simulink model "PIDQUAD_Position"  (R2016a)
settings: Solver=ode4  StartTime=0.0  StopTime=14  FixedStep=0.01  RelTol=1e-3
undefined symbols (not defined in the file): Disturbance, g, Ix, Iy, Iz, Jr, L, m, omega
libraries: simulink x7
settings Model: Creator=Morteza  LastModifiedBy=Novin Pendar

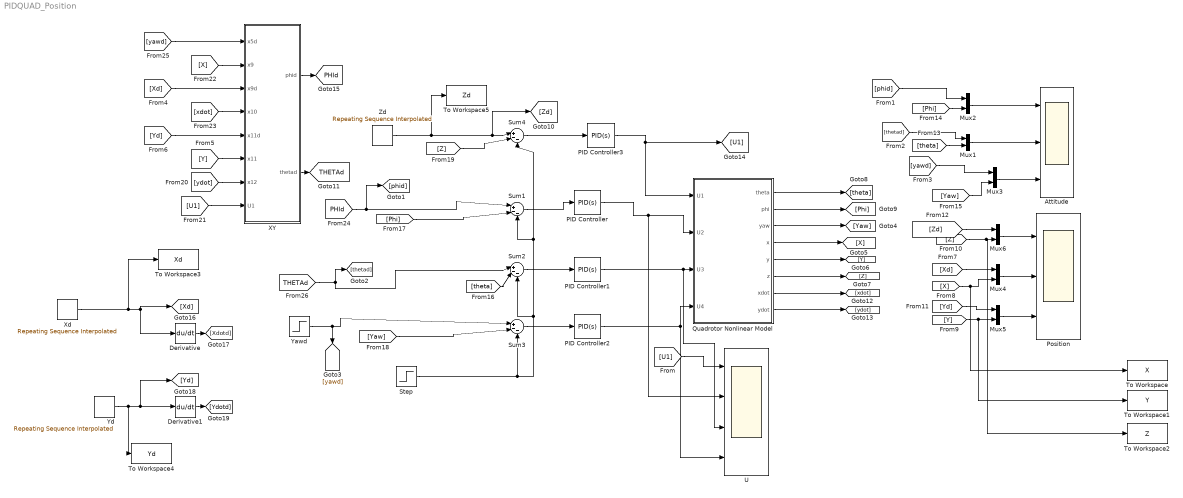
== system PIDQUAD_Position ==
  Attitude : Scope  NumInputPorts=3
  Derivative : Derivative
  Derivative1 : Derivative
  Mux{1..6} (6 alike) : Mux  Inputs=2
  PID Controller : simulink/Continuous/PID Controller  Controller=PID  TimeDomain=Continuous-time  SampleTime=-1  IntegratorMethod=Forward Euler  FilterMethod=Forward Euler  Form=Parallel  UseFilter=on  ControllerParametersSource=internal  P=5  I=1  D=0.199315858915149  N=100  InitialConditionSource=internal  InitialConditionForIntegrator=0  InitialConditionForFilter=0  ExternalReset=none  LimitOutput=off  UpperSaturationLimit=inf  LowerSaturationLimit=-inf  LinearizeAsGain=on  AntiWindupMode=none  Kb=1  TrackingMode=off  Kt=1  PParamMin=[]  PParamMax=[]  IParamMin=[]  IParamMax=[]  DParamMin=[]  DParamMax=[]  NParamMin=[]  NParamMax=[]  KbParamMin=[]  KbParamMax=[]  KtParamMin=[]  KtParamMax=[]  POutMin=[]  POutMax=[]  IOutMin=[]  IOutMax=[]  DOutMin=[]  DOutMax=[]  NOutMin=[]  NOutMax=[]  KbOutMin=[]  KbOutMax=[]  KtOutMin=[]  KtOutMax=[]  IntegratorOutMin=[]  IntegratorOutMax=[]  FilterOutMin=[]  FilterOutMax=[]  SumOutMin=[]  SumOutMax=[]  SumI1OutMin=[]  SumI1OutMax=[]  SumI2OutMin=[]  SumI2OutMax=[]  SumI3OutMin=[]  SumI3OutMax=[]  SumDOutMin=[]  SumDOutMax=[]  SaturationOutMin=[]  SaturationOutMax=[]  IntegratorContinuousStateAttributes=''  IntegratorStateMustResolveToSignalObject=off  IntegratorRTWStateStorageClass=Auto  FilterContinuousStateAttributes=''  FilterStateMustResolveToSignalObject=off  FilterRTWStateStorageClass=Auto  DifferentiatorICPrevScaledInput=0  DifferentiatorOutMin=[]  DifferentiatorOutMax=[]
  PID Controller1 : simulink/Continuous/PID Controller  Controller=PID  TimeDomain=Continuous-time  SampleTime=-1  IntegratorMethod=Forward Euler  FilterMethod=Forward Euler  Form=Parallel  UseFilter=on  ControllerParametersSource=internal  P=2  I=0.5  D=0.199315858915149  N=100  InitialConditionSource=internal  InitialConditionForIntegrator=0  InitialConditionForFilter=0  ExternalReset=none  LimitOutput=off  UpperSaturationLimit=inf  LowerSaturationLimit=-inf  LinearizeAsGain=on  AntiWindupMode=none  Kb=1  TrackingMode=off  Kt=1  PParamMin=[]  PParamMax=[]  IParamMin=[]  IParamMax=[]  DParamMin=[]  DParamMax=[]  NParamMin=[]  NParamMax=[]  KbParamMin=[]  KbParamMax=[]  KtParamMin=[]  KtParamMax=[]  POutMin=[]  POutMax=[]  IOutMin=[]  IOutMax=[]  DOutMin=[]  DOutMax=[]  NOutMin=[]  NOutMax=[]  KbOutMin=[]  KbOutMax=[]  KtOutMin=[]  KtOutMax=[]  IntegratorOutMin=[]  IntegratorOutMax=[]  FilterOutMin=[]  FilterOutMax=[]  SumOutMin=[]  SumOutMax=[]  SumI1OutMin=[]  SumI1OutMax=[]  SumI2OutMin=[]  SumI2OutMax=[]  SumI3OutMin=[]  SumI3OutMax=[]  SumDOutMin=[]  SumDOutMax=[]  SaturationOutMin=[]  SaturationOutMax=[]  IntegratorContinuousStateAttributes=''  IntegratorStateMustResolveToSignalObject=off  IntegratorRTWStateStorageClass=Auto  FilterContinuousStateAttributes=''  FilterStateMustResolveToSignalObject=off  FilterRTWStateStorageClass=Auto  DifferentiatorICPrevScaledInput=0  DifferentiatorOutMin=[]  DifferentiatorOutMax=[]
  PID Controller2 : simulink/Continuous/PID Controller  Controller=PID  TimeDomain=Continuous-time  SampleTime=-1  IntegratorMethod=Forward Euler  FilterMethod=Forward Euler  Form=Parallel  UseFilter=on  ControllerParametersSource=internal  P=0.417810086829264  I=0.2  D=0.347327554420679  N=34.4122258847421  InitialConditionSource=internal  InitialConditionForIntegrator=0  InitialConditionForFilter=0  ExternalReset=none  LimitOutput=off  UpperSaturationLimit=inf  LowerSaturationLimit=-inf  LinearizeAsGain=on  AntiWindupMode=none  Kb=1  TrackingMode=off  Kt=1  PParamMin=[]  PParamMax=[]  IParamMin=[]  IParamMax=[]  DParamMin=[]  DParamMax=[]  NParamMin=[]  NParamMax=[]  KbParamMin=[]  KbParamMax=[]  KtParamMin=[]  KtParamMax=[]  POutMin=[]  POutMax=[]  IOutMin=[]  IOutMax=[]  DOutMin=[]  DOutMax=[]  NOutMin=[]  NOutMax=[]  KbOutMin=[]  KbOutMax=[]  KtOutMin=[]  KtOutMax=[]  IntegratorOutMin=[]  IntegratorOutMax=[]  FilterOutMin=[]  FilterOutMax=[]  SumOutMin=[]  SumOutMax=[]  SumI1OutMin=[]  SumI1OutMax=[]  SumI2OutMin=[]  SumI2OutMax=[]  SumI3OutMin=[]  SumI3OutMax=[]  SumDOutMin=[]  SumDOutMax=[]  SaturationOutMin=[]  SaturationOutMax=[]  IntegratorContinuousStateAttributes=''  IntegratorStateMustResolveToSignalObject=off  IntegratorRTWStateStorageClass=Auto  FilterContinuousStateAttributes=''  FilterStateMustResolveToSignalObject=off  FilterRTWStateStorageClass=Auto  DifferentiatorICPrevScaledInput=0  DifferentiatorOutMin=[]  DifferentiatorOutMax=[]
  PID Controller3 : simulink/Continuous/PID Controller  Controller=PID  TimeDomain=Continuous-time  SampleTime=-1  IntegratorMethod=Forward Euler  FilterMethod=Forward Euler  Form=Parallel  UseFilter=on  ControllerParametersSource=internal  P=6  I=5  D=5  N=34.4122258847421  InitialConditionSource=internal  InitialConditionForIntegrator=0  InitialConditionForFilter=0  ExternalReset=none  LimitOutput=off  UpperSaturationLimit=inf  LowerSaturationLimit=-inf  LinearizeAsGain=on  AntiWindupMode=none  Kb=1  TrackingMode=off  Kt=1  PParamMin=[]  PParamMax=[]  IParamMin=[]  IParamMax=[]  DParamMin=[]  DParamMax=[]  NParamMin=[]  NParamMax=[]  KbParamMin=[]  KbParamMax=[]  KtParamMin=[]  KtParamMax=[]  POutMin=[]  POutMax=[]  IOutMin=[]  IOutMax=[]  DOutMin=[]  DOutMax=[]  NOutMin=[]  NOutMax=[]  KbOutMin=[]  KbOutMax=[]  KtOutMin=[]  KtOutMax=[]  IntegratorOutMin=[]  IntegratorOutMax=[]  FilterOutMin=[]  FilterOutMax=[]  SumOutMin=[]  SumOutMax=[]  SumI1OutMin=[]  SumI1OutMax=[]  SumI2OutMin=[]  SumI2OutMax=[]  SumI3OutMin=[]  SumI3OutMax=[]  SumDOutMin=[]  SumDOutMax=[]  SaturationOutMin=[]  SaturationOutMax=[]  IntegratorContinuousStateAttributes=''  IntegratorStateMustResolveToSignalObject=off  IntegratorRTWStateStorageClass=Auto  FilterContinuousStateAttributes=''  FilterStateMustResolveToSignalObject=off  FilterRTWStateStorageClass=Auto  DifferentiatorICPrevScaledInput=0  DifferentiatorOutMin=[]  DifferentiatorOutMax=[]
  Position : Scope  NumInputPorts=3
  Quadrotor Nonlinear Model : Subsystem
  Step : Step  Time=8  After=Disturbance  SampleTime=0
  Sum{1..4} (4 alike) : Sum  Inputs=|+--
  To Workspace : ToWorkspace  VariableName=X  SampleTime=-1
      settings: Save2DSignal=2-D array (concatenate along first dimension)
  To Workspace1 : ToWorkspace  VariableName=Y  SampleTime=-1
      settings: Save2DSignal=2-D array (concatenate along first dimension)
  To Workspace2 : ToWorkspace  VariableName=Z  SampleTime=-1
      settings: Save2DSignal=2-D array (concatenate along first dimension)
  To Workspace3 : ToWorkspace  VariableName=Xd  SampleTime=-1
      settings: Save2DSignal=2-D array (concatenate along first dimension)
  To Workspace4 : ToWorkspace  VariableName=Yd  SampleTime=-1
      settings: Save2DSignal=2-D array (concatenate along first dimension)
  To Workspace5 : ToWorkspace  VariableName=Zd  SampleTime=-1
      settings: Save2DSignal=2-D array (concatenate along first dimension)
  "U " : Scope  NumInputPorts=4
  XY : MATLAB Function  TreatAsAtomicUnit=on
  "Xd " : simulink/Sources/Repeating Sequence Interpolated  OutValues=[2 2 2 0 0].'  TimeValues="[0  3 6 9  14].'"  LookUpMeth=Interpolation-Use End Values  tsamp=0.01  OutMin=[]  OutMax=[]  OutDataTypeStr=double  OutputDataTypeScalingMode=double  OutDataType=fixdt(0,8)  OutScaling=2^-10
  Yawd : Step  Time=0  SampleTime=0
  "Yd " : simulink/Sources/Repeating Sequence Interpolated  OutValues=[2 2 5 5 0 0 ].'  TimeValues="[0 3  6 9 11 14].'"  LookUpMeth=Interpolation-Use End Values  tsamp=0.01  OutMin=[]  OutMax=[]  OutDataTypeStr=double  OutputDataTypeScalingMode=double  OutDataType=fixdt(0,8)  OutScaling=2^-10
  "Zd " : simulink/Sources/Repeating Sequence Interpolated  OutValues=[0.9 5 5].'  TimeValues="[0  3 14].'"  LookUpMeth=Interpolation-Use End Values  tsamp=0.01  OutMin=[]  OutMax=[]  OutDataTypeStr=double  OutputDataTypeScalingMode=double  OutDataType=fixdt(0,8)  OutScaling=2^-10
  tag scope: PHId=global, THETAd=global
  wires:
  Mux3/1 -> Attitude/3
  [thetad] -> Mux1/1
  [yawd] -> Mux3/1
  Quadrotor Nonlinear Model/5(y) -> [Y]
  Quadrotor Nonlinear Model/6(z) -> [Z]
  Quadrotor Nonlinear Model/4(x) -> [X]
  Quadrotor Nonlinear Model/3(yaw) -> [Yaw]
  Quadrotor Nonlinear Model/2(phi) -> [Phi]
  Quadrotor Nonlinear Model/1(theta) -> [theta]
  [Z] -> To Workspace2/1, Mux6/2
  [Y] -> To Workspace1/1, Mux5/2
  [X] -> To Workspace/1, Mux4/2
  [Zd] -> Mux6/1
  [Yd] -> Mux5/1
  [Xd] -> Mux4/1
  [theta] -> Mux1/2
  [Phi] -> Mux2/2
  [Yaw] -> Mux3/2
  Yawd/1 -> Sum3/1, [yawd]
  [Yaw] -> Sum3/2
  Sum1/1 -> PID Controller/1
  Sum2/1 -> PID Controller1/1
  Sum3/1 -> PID Controller2/1
  PID Controller/1 -> Quadrotor Nonlinear Model/2(U2), "U "/2
  PID Controller1/1 -> "U "/3, Quadrotor Nonlinear Model/3(U3)
  PID Controller2/1 -> Quadrotor Nonlinear Model/4(U4), "U "/4
  "Zd "/1 -> To Workspace5/1, [Zd], Sum4/1
  [Z] -> Sum4/2
  Sum4/1 -> PID Controller3/1
  PID Controller3/1 -> Quadrotor Nonlinear Model/1(U1), [U1]
  Mux1/1 -> Attitude/2
  Mux2/1 -> Attitude/1
  [Phi] -> Sum1/2
  [theta] -> Sum2/2
  Mux6/1 -> Position/1
  Mux4/1 -> Position/2
  Mux5/1 -> Position/3
  Quadrotor Nonlinear Model/7(xdot) -> [xdot]
  Quadrotor Nonlinear Model/8(ydot) -> [ydot]
  [THETAd] -> [thetad], Sum2/1
  [U1] -> "U "/1
  [phid] -> Mux2/1
  [X] -> XY/2(x9)
  [Xd] -> XY/3(x9d)
  [xdot] -> XY/4(x10)
  [Yd] -> XY/5(x11d)
  [Y] -> XY/6(x11)
  [ydot] -> XY/7(x12)
  [U1] -> XY/8(U1)
  XY/1(phid) -> [PHId]
  XY/2(thetad) -> [THETAd]
  [yawd] -> XY/1(x5d)
  "Xd "/1 -> To Workspace3/1, Derivative/1, [Xd]
  Derivative/1 -> [Xdotd]
  "Yd "/1 -> To Workspace4/1, [Yd], Derivative1/1
  Derivative1/1 -> [Ydotd]
  [PHId] -> Sum1/1, [phid]
  Step/1 -> Sum4/3, Sum1/3, Sum2/3, Sum3/3

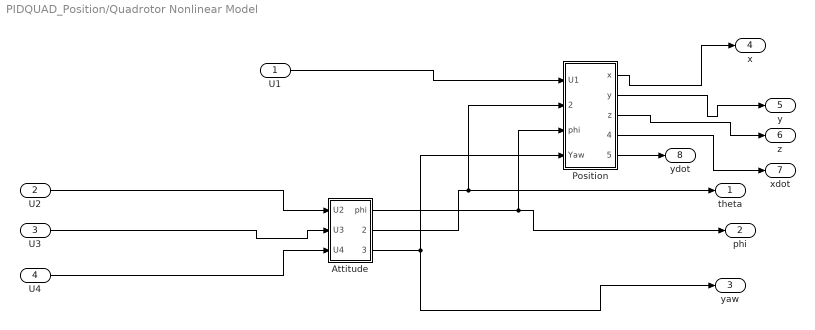
== system PIDQUAD_Position/Quadrotor Nonlinear Model ==
  U1 : Inport
  U2 : Inport  Port=2
  U3 : Inport  Port=3
  U4 : Inport  Port=4
  "Attitude " : Subsystem
  Position : Subsystem
  theta : Outport
  phi : Outport  Port=2
  yaw : Outport  Port=3
  x : Outport  Port=4
  y : Outport  Port=5
  z : Outport  Port=6
  xdot : Outport  Port=7
  ydot : Outport  Port=8
  wires:
  Position/2(y) -> y/1
  Position/3(z) -> z/1
  Position/1(x) -> x/1
  U3/1 -> "Attitude "/2(U3)
  U4/1 -> "Attitude "/3(U4)
  U2/1 -> "Attitude "/1(U2)
  "Attitude "/2(theta) -> Position/2(Theta), theta/1
  "Attitude "/1("phi ") -> Position/3(phi), phi/1
  U1/1 -> Position/1(U1)
  Position/4(xdot) -> xdot/1
  Position/5(ydot) -> ydot/1
  "Attitude "/3(yaw) -> yaw/1, Position/4(Yaw)

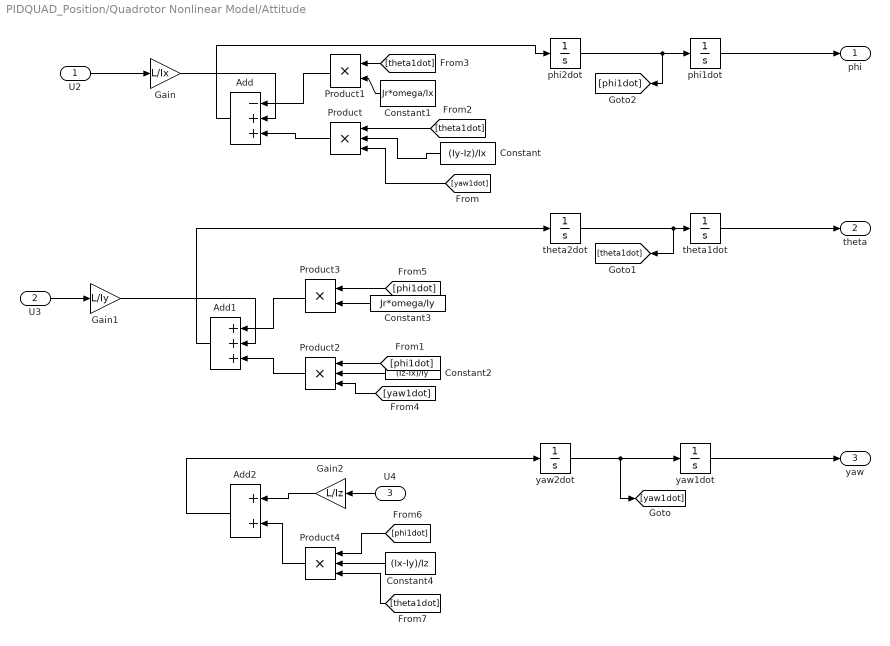
== system PIDQUAD_Position/Quadrotor Nonlinear Model/Attitude  ==
  U2 : Inport
  U3 : Inport  Port=2
  U4 : Inport  Port=3
  Add : Sum  Inputs=-++
  Add1 : Sum  Inputs=+++
  Add2 : Sum
  Constant : Constant  Value=(Iy-Iz)/Ix
  Constant1 : Constant  Value=Jr*omega/Ix
  Constant2 : Constant  Value=(Iz-Ix)/Iy
  Constant3 : Constant  Value=Jr*omega/Iy
  Constant4 : Constant  Value=(Ix-Iy)/Iz
  Gain : Gain  Gain=L/Ix
  Gain1 : Gain  Gain=L/Iy
  Gain2 : Gain  Gain=L/Iz
  Product : Product  Inputs=3
  Product1 : Product
  Product2 : Product  Inputs=3
  Product3 : Product
  Product4 : Product  Inputs=3
  phi1dot : Integrator
  phi2dot : Integrator
  theta1dot : Integrator
  theta2dot : Integrator
  yaw1dot : Integrator
  yaw2dot : Integrator
  "phi " : Outport
  theta : Outport  Port=2
  yaw : Outport  Port=3
  wires:
  theta2dot/1 -> [theta1dot], theta1dot/1
  Product/1 -> Add/3
  phi2dot/1 -> [phi1dot], phi1dot/1
  U2/1 -> Gain/1
  Add/1 -> phi2dot/1
  Product3/1 -> Add1/1
  [phi1dot] -> Product3/1
  Constant3/1 -> Product3/2
  U4/1 -> Gain2/1
  Product4/1 -> Add2/2
  Constant/1 -> Product/2
  Gain/1 -> Add/2
  phi1dot/1 -> "phi "/1
  yaw2dot/1 -> [yaw1dot], yaw1dot/1
  yaw1dot/1 -> yaw/1
  [yaw1dot] -> Product2/3
  Constant2/1 -> Product2/2
  [phi1dot] -> Product2/1
  Add2/1 -> yaw2dot/1
  Gain2/1 -> Add2/1
  [phi1dot] -> Product4/1
  [theta1dot] -> Product4/3
  Constant4/1 -> Product4/2
  Product2/1 -> Add1/3
  Product1/1 -> Add/1
  Add1/1 -> theta2dot/1
  U3/1 -> Gain1/1
  Gain1/1 -> Add1/2
  theta1dot/1 -> theta/1
  [theta1dot] -> Product/1
  [yaw1dot] -> Product/3
  Constant1/1 -> Product1/2
  [theta1dot] -> Product1/1

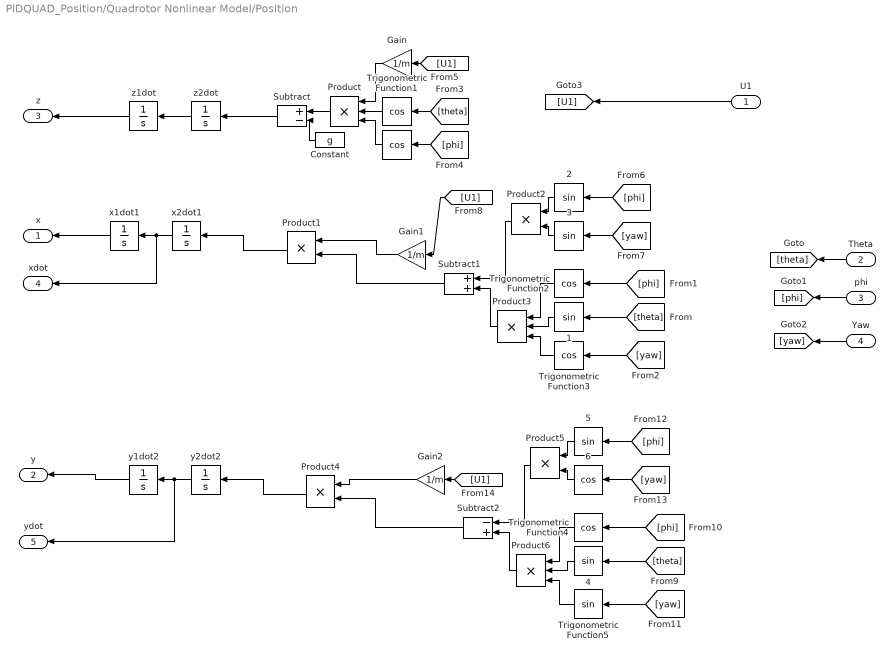
== system PIDQUAD_Position/Quadrotor Nonlinear Model/Position ==
  U1 : Inport
  Theta : Inport  Port=2
  phi : Inport  Port=3
  Yaw : Inport  Port=4
  " " : Trigonometry  Operator=cos
   {1..5} (5 alike) : Trigonometry
  " 6" : Trigonometry  Operator=cos
  Constant : Constant  Value=g
  Gain : Gain  Gain=1/m
  Gain1 : Gain  Gain=1/m
  Gain2 : Gain  Gain=1/m
  Product : Product  Inputs=3
  Product{1..2,4..5} (4 alike) : Product
  Product3 : Product  Inputs=3
  Product6 : Product  Inputs=3
  Subtract : Sum  Inputs=+-
  Subtract1 : Sum
  Subtract2 : Sum  Inputs=-+
  Trigonometric Function{1..4} (4 alike) : Trigonometry  Operator=cos
  Trigonometric Function5 : Trigonometry
  x1dot1 : Integrator  InitialCondition=2
  x2dot1 : Integrator
  y1dot2 : Integrator  InitialCondition=2
  y2dot2 : Integrator
  z1dot : Integrator  InitialCondition=1
  z2dot : Integrator
  x : Outport
  y : Outport  Port=2
  z : Outport  Port=3
  xdot : Outport  Port=4
  ydot : Outport  Port=5
  wires:
  Subtract1/1 -> Product1/2
  Gain/1 -> Product/1
  y1dot2/1 -> y/1
  Product1/1 -> x2dot1/1
  x1dot1/1 -> x/1
  [yaw] -> Trigonometric Function5/1
  " "/1 -> Product/3
  [yaw] -> Trigonometric Function3/1
  Trigonometric Function1/1 -> Product/2
  [yaw] -> " 3"/1
  [phi] -> Trigonometric Function2/1
  Product3/1 -> Subtract1/2
  Product/1 -> Subtract/1
  [U1] -> Gain2/1
  Product5/1 -> Subtract2/1
  [phi] -> Trigonometric Function4/1
  [yaw] -> " 6"/1
  Gain2/1 -> Product4/1
  Trigonometric Function4/1 -> Product6/1
  " 4"/1 -> Product6/2
  Subtract2/1 -> Product4/2
  [theta] -> " 4"/1
  " 5"/1 -> Product5/1
  Trigonometric Function5/1 -> Product6/3
  " 6"/1 -> Product5/2
  Product6/1 -> Subtract2/2
  y2dot2/1 -> ydot/1, y1dot2/1
  [phi] -> " 5"/1
  Product4/1 -> y2dot2/1
  [U1] -> Gain/1
  [U1] -> Gain1/1
  [theta] -> " 1"/1
  z1dot/1 -> z/1
  Gain1/1 -> Product1/1
  Trigonometric Function2/1 -> Product3/1
  [phi] -> " 2"/1
  " 1"/1 -> Product3/2
  z2dot/1 -> z1dot/1
  U1/1 -> [U1]
  [theta] -> Trigonometric Function1/1
  [phi] -> " "/1
  Constant/1 -> Subtract/2
  Trigonometric Function3/1 -> Product3/3
  x2dot1/1 -> xdot/1, x1dot1/1
  " 3"/1 -> Product2/2
  Subtract/1 -> z2dot/1
  Product2/1 -> Subtract1/1
  " 2"/1 -> Product2/1
  Theta/1 -> [theta]
  phi/1 -> [phi]
  Yaw/1 -> [yaw]

== matlab function PIDQUAD_Position/XY ==
  data: phid output; x5d input; x9 input; x9d input; x10 input; x11d input; x11 input; x12 input; U1 input; thetad output
function [phid,thetad ]= XY(x5d,x9,x9d,x10,x11d,x11,x12,U1)
m=0.65;
k1=8;
k2=5;
k3=6;
k4=4;

ux = (m/U1)*(k1*(x9d-x9)-k2*x10);
uy=(m/U1)*(k3*(x11d-x11)-k4*x12);
phid=real(asin(complex(sin(x5d)*ux-cos(x5d)*uy)));
thetad=real(asin(complex((cos(x5d)*ux+sin(x5d)*uy)/cos(phid))));
